simulink model "PMLSM_ThreeLoop_Simple"  (R2026a)
settings: Solver=FixedStepDiscrete  StopTime=12  FixedStep=PMLSM_Ts_s
InitFcn:
  | reload(get_param('PMLSM_ThreeLoop_Simple','ModelWorkspace'));
model workspace: external: MATLAB File init_PMLSM_ThreeLoop_Simple.m (data not in the file)
values from neighbouring files (symbols this model uses):
  CPU_Clock = 200e6    (= 200000000)    [PMSLM_Init_Params_MBDL4.m]    (also in init_PMLSM_ThreeLoop_Simple.m)
  Host_Enable_Schedule = [0 1 1 1]    [init_PMLSM_ThreeLoop_Simple.m]
  Host_Id_A = 0    [init_PMLSM_ThreeLoop_Simple.m]
  Host_Iq_A = 0    [init_PMLSM_ThreeLoop_Simple.m]
  Host_Iq_Test_Mode = 0    [init_PMLSM_ThreeLoop_Simple.m]
  Host_Load_N = 0    [init_PMLSM_ThreeLoop_Simple.m]
  Host_PI_Reset_EN = 0    [init_PMLSM_ThreeLoop_Simple.m]
  Host_Speed_mmps = 0    [init_PMLSM_ThreeLoop_Simple.m]
  Host_Speed_Ramp_s = 1    [init_PMLSM_ThreeLoop_Simple.m]
  Host_Start_s = 0.5    [init_PMLSM_ThreeLoop_Simple.m]
  Host_Target_mm = 100    [init_PMLSM_ThreeLoop_Simple.m]
  Host_Traj_Amax = 100    [init_PMLSM_ThreeLoop_Simple.m]
  Host_Traj_Jmax = 1000    [init_PMLSM_ThreeLoop_Simple.m]
  Host_Traj_Vmax = 20    [init_PMLSM_ThreeLoop_Simple.m]
  Iq_fric_run = 0.05    [PMSLM_Init_Params_MBDL4.m]
  Iq_fric_start = 0.40    (= 0.4)    [PMSLM_Init_Params_MBDL4.m]
  Iq_int_limit = 0.10    (= 0.1)    [PMSLM_Init_Params_MBDL4.m]    (also in init_PMLSM_ThreeLoop_Simple.m = 0.5)
  Kaw_d = Kaw_q    (= 0.2)    [PMSLM_Init_Params_MBDL4.m]    (also in init_PMLSM_ThreeLoop_Simple.m = Tuning_Gains.Kaw_d)
  Kaw_q = 0.2    [PMSLM_Init_Params_MBDL4.m]    (also in init_PMLSM_ThreeLoop_Simple.m = Tuning_Gains.Kaw_q)
  Kaw_s = 0.4    [PMSLM_Init_Params_MBDL4.m]    (also in init_PMLSM_ThreeLoop_Simple.m = Tuning_Gains.Kaw_s)
  Ki_ACR = ACR_Commissioning_Scale*Ki_ACR_Baseline    (= 2962.5)    [PMSLM_Init_Params_MBDL4.m]    (also in init_PMLSM_ThreeLoop_Simple.m = Tuning_Gains.Ki_ACR; init_PMLSM_mil_test_params.m = Kp_ACR*PMLSM_Rs_ohm/PMLSM_Lq_H)
  Ki_ASR = 0.05    [PMSLM_Init_Params_MBDL4.m]    (also in init_PMLSM_ThreeLoop_Simple.m = Tuning_Gains.Ki_ASR)
  Kp_ACR = ACR_Commissioning_Scale*Kp_ACR_Baseline    (= 2.18125)    [PMSLM_Init_Params_MBDL4.m]    (also in init_PMLSM_ThreeLoop_Simple.m = Tuning_Gains.Kp_ACR; init_PMLSM_mil_test_params.m = PMLSM_Lq_H/(4*MIL_AUM3S4_Current_PI_xi^2*MIL_AUM3S4_Current_)
  Kp_ASR = 0.03    [PMSLM_Init_Params_MBDL4.m]    (also in init_PMLSM_ThreeLoop_Simple.m = Tuning_Gains.Kp_ASR)
  Kp_pos = 5    [PMSLM_Init_Params_MBDL4.m]    (also in init_PMLSM_ThreeLoop_Simple.m = Tuning_Gains.Kp_pos)
  PMLSM_Bv_N_per_mps = 0    [init_PMLSM_ThreeLoop_Simple.m]    (also in init_PMLSM_plant_params.m)
  PMLSM_deadtime_current_eps_A = 1e-4    (= 0.0001)    [init_PMLSM_ThreeLoop_Simple.m]    (also in init_PMLSM_plant_params.m)
  PMLSM_deadtime_ratio = PMLSM_deadtime_s/Ts    (= 0.01)    [init_PMLSM_ThreeLoop_Simple.m]    (also in init_PMLSM_plant_params.m)
  PMLSM_Fc_N = 0    [init_PMLSM_ThreeLoop_Simple.m]    (also in init_PMLSM_plant_params.m)
  PMLSM_Kf_peak_N_per_Apeak = 31.4/sqrt(2)    [init_PMLSM_ThreeLoop_Simple.m]    (also in init_PMLSM_plant_params.m = PMLSM_Kf_rms_N_per_Arms/sqrt(2))
  PMLSM_Ld_H = Ld    (= 0.001745)    [PMSLM_Init_Params_MBDL4.m]    (also in init_PMLSM_ThreeLoop_Simple.m; init_PMLSM_plant_params.m)
  PMLSM_Lq_H = Lq    (= 0.001745)    [PMSLM_Init_Params_MBDL4.m]    (also in init_PMLSM_ThreeLoop_Simple.m; init_PMLSM_plant_params.m)
  PMLSM_M_kg = 0.91    [init_PMLSM_ThreeLoop_Simple.m]    (also in init_PMLSM_plant_params.m)
  PMLSM_psi_f_Wb = flux    (= 0.141)    [PMSLM_Init_Params_MBDL4.m]    (also in init_PMLSM_ThreeLoop_Simple.m; init_PMLSM_plant_params.m)
  PMLSM_pwm_period_counts = CPU_Clock*Ts/2    (= 10000)    [init_PMLSM_ThreeLoop_Simple.m]    (also in init_PMLSM_plant_params.m = 7500)
  PMLSM_Rs_ohm = Rs    (= 2.37)    [PMSLM_Init_Params_MBDL4.m]    (also in init_PMLSM_ThreeLoop_Simple.m; init_PMLSM_plant_params.m)
  PMLSM_tau_NN_m = 0.06    [init_PMLSM_ThreeLoop_Simple.m]    (also in init_PMLSM_plant_params.m)
  PMLSM_theta_offset_rad = 0    [init_PMLSM_ThreeLoop_Simple.m]    (also in init_PMLSM_plant_params.m)
  PMLSM_Ts_s = Ts/2    (= 5e-05)    [init_PMLSM_ThreeLoop_Simple.m]    (also in init_PMLSM_plant_params.m = 0.0001)
  PMLSM_v_eps_mps = 1e-3    (= 0.001)    [init_PMLSM_ThreeLoop_Simple.m]    (also in init_PMLSM_plant_params.m)
  Pos_deadband = 0.02    [PMSLM_Init_Params_MBDL4.m]    (also in init_PMLSM_ThreeLoop_Simple.m)
  Speed_loop_Iq_Limit = Iq_Limit    (= 0.3)    [PMSLM_Init_Params_MBDL4.m]    (also in init_PMLSM_ThreeLoop_Simple.m = 1)
  Ts = 1 / PWM_Freq    (= 0.0001)    [PMSLM_Init_Params_MBDL4.m]    (also in init_PMLSM_ThreeLoop_Simple.m)
  Ts_ACR = 1e-4    (= 0.0001)    [PMSLM_Init_Params_MBDL4.m]    (also in init_PMLSM_ThreeLoop_Simple.m)
  Ts_ASR = 1e-3    (= 0.001)    [PMSLM_Init_Params_MBDL4.m]    (also in init_PMLSM_ThreeLoop_Simple.m)
  Udc = 48    [PMSLM_Init_Params_MBDL4.m]    (also in init_PMLSM_ThreeLoop_Simple.m; init_PMLSM_mil_test_params.m)
  v_ff_eps = 0.5    [PMSLM_Init_Params_MBDL4.m]    (also in init_PMLSM_ThreeLoop_Simple.m)
  v_over_eps = 3    [PMSLM_Init_Params_MBDL4.m]    (also in init_PMLSM_ThreeLoop_Simple.m)
  V_pos_max_mmps = 10    [PMSLM_Init_Params_MBDL4.m]    (also in init_PMLSM_ThreeLoop_Simple.m = 20)
  v_ref_max = 20    [PMSLM_Init_Params_MBDL4.m]    (also in init_PMLSM_ThreeLoop_Simple.m)
  v_ref_set_step_dn = v_ref_set_rate_dn * Ts    (= 0.005)    [PMSLM_Init_Params_MBDL4.m]    (also in init_PMLSM_ThreeLoop_Simple.m)
  v_ref_set_step_up = v_ref_set_rate_up * Ts    (= 0.005)    [PMSLM_Init_Params_MBDL4.m]    (also in init_PMLSM_ThreeLoop_Simple.m)
  v_ref_zero_eps = 0.2    [PMSLM_Init_Params_MBDL4.m]    (also in init_PMLSM_ThreeLoop_Simple.m = 0)
  v_stick_off = 3.0    (= 3)    [PMSLM_Init_Params_MBDL4.m]
  v_stick_on = 1.0    (= 1)    [PMSLM_Init_Params_MBDL4.m]
undefined symbols (not defined in the file or in its folder): DiscIntNeverNeededParam
libraries: simulink x7, mcbeeMathTransformLib x2
settings Model: Creator=lww  LastModifiedBy=lww

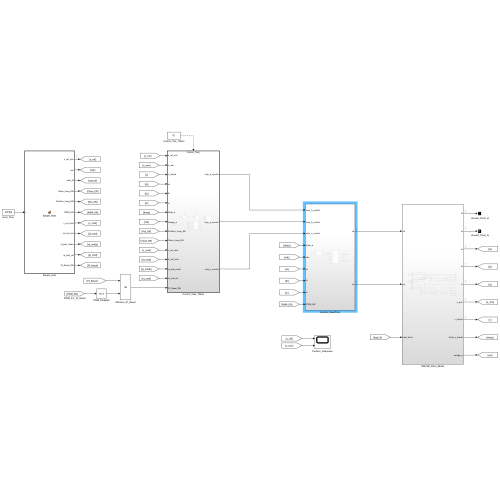
[thumbnail: Simulink's stored preview of the top-level diagram]
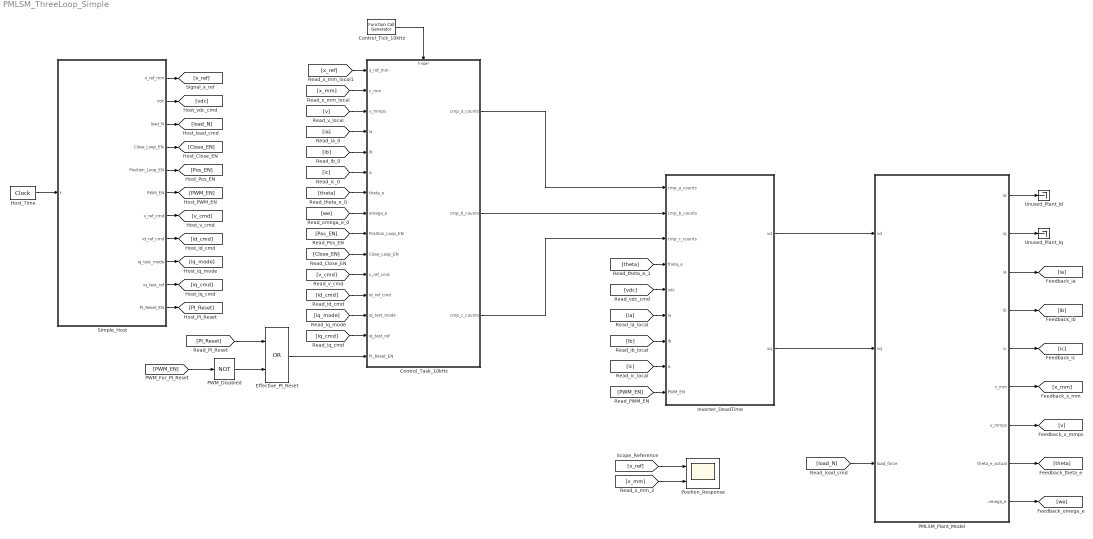
== system PMLSM_ThreeLoop_Simple ==
  Control_Task_10kHz : Subsystem
  Control_Tick_10kHz : FunctionCallGenerator  SampleTime=Ts
  Effective_PI_Reset : Logic  Operator=OR  AllPortsSameDT=off  OutDataTypeStr=boolean
  Host_Time : DigitalClock  SampleTime=Ts_ACR
  Inverter_DeadTime : Subsystem
  PMLSM_Plant_Model : Subsystem
  PWM_Disabled : Logic  Operator=NOT  AllPortsSameDT=off  OutDataTypeStr=boolean
  Position_Response : Scope  NumInputPorts=2
  Simple_Host : MATLAB Function  TreatAsAtomicUnit=on
  Unused_Plant_Id : Terminator
  Unused_Plant_Iq : Terminator
  wires:
  Host_Time/1 -> Simple_Host/1(t)
  [x_ref] -> Position_Response/1
  [ic] -> Inverter_DeadTime/8(ic)
  [ib] -> Inverter_DeadTime/7(ib)
  [ia] -> Inverter_DeadTime/6(ia)
  [x_mm] -> Position_Response/2
  [theta] -> Inverter_DeadTime/4(theta_e)
  [load_N] -> PMLSM_Plant_Model/3(load_force)
  [vdc] -> Inverter_DeadTime/5(vdc)
  Simple_Host/2(vdc) -> [vdc]
  Inverter_DeadTime/1(vd) -> PMLSM_Plant_Model/1(vd)
  Inverter_DeadTime/2(vq) -> PMLSM_Plant_Model/2(vq)
  PMLSM_Plant_Model/2(iq) -> Unused_Plant_Iq/1
  PMLSM_Plant_Model/1(id) -> Unused_Plant_Id/1
  PMLSM_Plant_Model/9(omega_e) -> [we]
  PMLSM_Plant_Model/8(theta_e_actual) -> [theta]
  PMLSM_Plant_Model/5(ic) -> [ic]
  PMLSM_Plant_Model/4(ib) -> [ib]
  PMLSM_Plant_Model/3(ia) -> [ia]
  PMLSM_Plant_Model/7(v_mmps) -> [v]
  PMLSM_Plant_Model/6(x_mm) -> [x_mm]
  Simple_Host/3(load_N) -> [load_N]
  Simple_Host/11(PI_Reset_EN) -> [PI_Reset]
  Simple_Host/10(iq_test_ref) -> [iq_cmd]
  Simple_Host/9(iq_test_mode) -> [iq_mode]
  Simple_Host/8(id_ref_cmd) -> [id_cmd]
  Simple_Host/7(v_ref_cmd) -> [v_cmd]
  [PWM_EN] -> Inverter_DeadTime/9(PWM_EN)
  Simple_Host/6(PWM_EN) -> [PWM_EN]
  Simple_Host/5(Position_Loop_EN) -> [Pos_EN]
  Simple_Host/4(Close_Loop_EN) -> [Close_EN]
  [PWM_EN] -> PWM_Disabled/1
  PWM_Disabled/1 -> Effective_PI_Reset/2
  Effective_PI_Reset/1 -> Control_Task_10kHz/15(PI_Reset_EN)
  [Close_EN] -> Control_Task_10kHz/10(Close_Loop_EN)
  [Pos_EN] -> Control_Task_10kHz/9(Position_Loop_EN)
  [v_cmd] -> Control_Task_10kHz/11(v_ref_cmd)
  [id_cmd] -> Control_Task_10kHz/12(id_ref_cmd)
  [iq_mode] -> Control_Task_10kHz/13(iq_test_mode)
  [iq_cmd] -> Control_Task_10kHz/14(iq_test_ref)
  [PI_Reset] -> Effective_PI_Reset/1
  Simple_Host/1(x_ref_mm) -> [x_ref]
  Control_Task_10kHz/1(cmp_a_counts) -> Inverter_DeadTime/1(cmp_a_counts)
  Control_Task_10kHz/2(cmp_b_counts) -> Inverter_DeadTime/2(cmp_b_counts)
  Control_Task_10kHz/3(cmp_c_counts) -> Inverter_DeadTime/3(cmp_c_counts)
  [x_mm] -> Control_Task_10kHz/2(x_mm)
  [v] -> Control_Task_10kHz/3(v_mmps)
  [ia] -> Control_Task_10kHz/4(ia)
  [ib] -> Control_Task_10kHz/5(ib)
  [ic] -> Control_Task_10kHz/6(ic)
  [we] -> Control_Task_10kHz/8(omega_e)
  [theta] -> Control_Task_10kHz/7(theta_e)
  Control_Tick_10kHz/1 -> Control_Task_10kHz/Trigger
  [x_ref] -> Control_Task_10kHz/1(x_ref_mm)

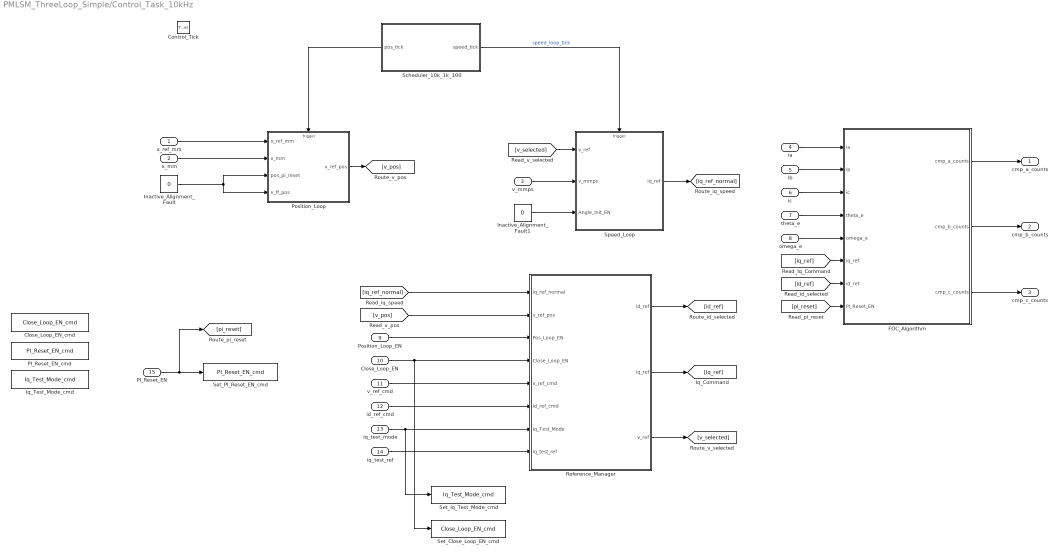
== system PMLSM_ThreeLoop_Simple/Control_Task_10kHz ==
  x_ref_mm : Inport
  x_mm : Inport  Port=2
  v_mmps : Inport  Port=3
  ia : Inport  Port=4
  ib : Inport  Port=5
  ic : Inport  Port=6
  theta_e : Inport  Port=7
  omega_e : Inport  Port=8
  Position_Loop_EN : Inport  Port=9
  Close_Loop_EN : Inport  Port=10
  v_ref_cmd : Inport  Port=11
  id_ref_cmd : Inport  Port=12
  iq_test_mode : Inport  Port=13
  iq_test_ref : Inport  Port=14
  PI_Reset_EN : Inport  Port=15
  Control_Tick : TriggerPort  TriggerType=function-call  VariantControl=(inherit)  PortDimensions=1
  Close_Loop_EN_cmd : DataStoreMemory  DataStoreName=Close_Loop_EN_cmd  WriteAfterWriteMsg=warning  InitialValue=1  ShowAdditionalParam=off
  FOC_Algorithm : Subsystem
  Inactive_Alignment_Fault : Constant  Value=0
  Inactive_Alignment_Fault1 : Constant  Value=0
  Iq_Test_Mode_cmd : DataStoreMemory  DataStoreName=Iq_Test_Mode_cmd  WriteAfterWriteMsg=warning  ShowAdditionalParam=off
  PI_Reset_EN_cmd : DataStoreMemory  DataStoreName=PI_Reset_EN_cmd  WriteAfterWriteMsg=warning  ShowAdditionalParam=off
  Position_Loop : Subsystem  TreatAsAtomicUnit=on
  Reference_Manager : Subsystem
  Scheduler_10k_1k_100 : Subsystem
      settings: PortSchema="{\"entries\":[{\"content\":{\"sides\":[{\"content\":{\"connectorIds\":[\"Out2\"]},\"type\":\"ConnectorPlacement.EquallySpacedRectSide\",\"uuid\":\"7a2cd2ad-1b6d-4ced-b4c0-dea2e76e4441\"},{\"content\":{\"connectorIds\":[\"Out1\"],\"side\":\"RIGHT\"},\"type\":\"ConnectorPlacement.EquallySpacedRectSide\",\"uuid\":\"f7db3b94-1126-4089-83bd-8e57d20e6fd7\"},{\"content\":{\"side\":\"TOP\"},\"type\":\"ConnectorPlacement.EquallySpacedRectSide\",\"uuid\":\"9153f6b5-22af-48be-92c0-68be43f93648\"}]},\"type\":\"ConnectorPlacement.EquallySpacedConnector\",\"uuid\":\"029fb485-bddc-4cd2-9c64-7547c8dffd2b\"}],\"packageUris\":[\"http://schema.mathworks.com/mf0/Connector/R2020b\"],\"version\":\"1.0\"}"
  Set_Close_Loop_EN_cmd : DataStoreWrite  Priority=-10  DataStoreName=Close_Loop_EN_cmd  IndexOptions=Index vector (dialog)  Indices=1  OutputSizes=1
  Set_Iq_Test_Mode_cmd : DataStoreWrite  Priority=-10  DataStoreName=Iq_Test_Mode_cmd  IndexOptions=Index vector (dialog)  Indices=1  OutputSizes=1
  Set_PI_Reset_EN_cmd : DataStoreWrite  Priority=-10  DataStoreName=PI_Reset_EN_cmd  IndexOptions=Index vector (dialog)  Indices=1  OutputSizes=1
  Speed_Loop : Subsystem  TreatAsAtomicUnit=on
  cmp_a_counts : Outport
  cmp_b_counts : Outport  Port=2
  cmp_c_counts : Outport  Port=3
  wires:
  [iq_ref] -> FOC_Algorithm/6(iq_ref)
  FOC_Algorithm/3(cmp_c_counts) -> cmp_c_counts/1
  FOC_Algorithm/2(cmp_b_counts) -> cmp_b_counts/1
  FOC_Algorithm/1(cmp_a_counts) -> cmp_a_counts/1
  omega_e/1 -> FOC_Algorithm/5(omega_e)
  theta_e/1 -> FOC_Algorithm/4(theta_e)
  ic/1 -> FOC_Algorithm/3(ic)
  ib/1 -> FOC_Algorithm/2(ib)
  ia/1 -> FOC_Algorithm/1(ia)
  Reference_Manager/2(iq_ref) -> [iq_ref]
  iq_test_ref/1 -> Reference_Manager/8(iq_test_ref)
  id_ref_cmd/1 -> Reference_Manager/6(id_ref_cmd)
  v_ref_cmd/1 -> Reference_Manager/5(v_ref_cmd)
  Position_Loop_EN/1 -> Reference_Manager/3(Pos_Loop_EN)
  [pi_reset] -> FOC_Algorithm/8(PI_Reset_EN)
  [id_ref] -> FOC_Algorithm/7(id_ref)
  [v_selected] -> Speed_Loop/1(v_ref)
  [iq_ref_normal] -> Reference_Manager/1(iq_ref_normal)
  [v_pos] -> Reference_Manager/2(v_ref_pos)
  Reference_Manager/3(v_ref) -> [v_selected]
  Inactive_Alignment_Fault/1 -> Position_Loop/3(pos_pi_reset), Position_Loop/4(v_ff_pos)
  Speed_Loop/1(iq_ref) -> [iq_ref_normal]
  Position_Loop/1(v_ref_pos) -> [v_pos]
  x_mm/1 -> Position_Loop/2(x_mm)
  x_ref_mm/1 -> Position_Loop/1(x_ref_mm)
  Scheduler_10k_1k_100/1(speed_tick) -> Speed_Loop/Trigger  "speed_loop_tick"
  Scheduler_10k_1k_100/2(pos_tick) -> Position_Loop/Trigger
  PI_Reset_EN/1 -> [pi_reset], Set_PI_Reset_EN_cmd/1
  Reference_Manager/1(id_ref) -> [id_ref]
  iq_test_mode/1 -> Set_Iq_Test_Mode_cmd/1, Reference_Manager/7(Iq_Test_Mode)
  Close_Loop_EN/1 -> Set_Close_Loop_EN_cmd/1, Reference_Manager/4(Close_Loop_EN)
  Inactive_Alignment_Fault1/1 -> Speed_Loop/3(Angle_Init_EN)
  v_mmps/1 -> Speed_Loop/2(v_mmps)

== system PMLSM_ThreeLoop_Simple/Inverter_DeadTime ==
  note: 死区时间建立
  note: 半拍更新延迟
  cmp_a_counts : Inport
  cmp_b_counts : Inport  Port=2
  cmp_c_counts : Inport  Port=3
  theta_e : Inport  Port=4
  vdc : Inport  Port=5
  ia : Inport  Port=6
  ib : Inport  Port=7
  ic : Inport  Port=8
  PWM_EN : Inport  Port=9
  DeadTime_Voltage_Model : Subsystem
  PWM_Update_HalfTs : Subsystem
  vd_PWM_Enable : Product  Inputs=**
  vq_PWM_Enable : Product  Inputs=**
  vd : Outport
  vq : Outport  Port=2
  wires:
  cmp_c_counts/1 -> PWM_Update_HalfTs/3(duty_c)
  cmp_b_counts/1 -> PWM_Update_HalfTs/2(duty_b)
  cmp_a_counts/1 -> PWM_Update_HalfTs/1(duty_a)
  vq_PWM_Enable/1 -> vq/1
  vd_PWM_Enable/1 -> vd/1
  PWM_Update_HalfTs/1(duty_a_delayed) -> DeadTime_Voltage_Model/1(duty_a)
  PWM_Update_HalfTs/2(duty_b_delayed) -> DeadTime_Voltage_Model/2(duty_b)
  PWM_Update_HalfTs/3(duty_c_delayed) -> DeadTime_Voltage_Model/3(duty_c)
  theta_e/1 -> DeadTime_Voltage_Model/4(theta_e)
  vdc/1 -> DeadTime_Voltage_Model/5(vdc)
  ia/1 -> DeadTime_Voltage_Model/6(ia_phase)
  ib/1 -> DeadTime_Voltage_Model/7(ib_phase)
  ic/1 -> DeadTime_Voltage_Model/8(ic_phase)
  DeadTime_Voltage_Model/1(vd_from_duty) -> vd_PWM_Enable/1
  DeadTime_Voltage_Model/2(vq_from_duty) -> vq_PWM_Enable/1
  PWM_EN/1 -> vd_PWM_Enable/2, vq_PWM_Enable/2

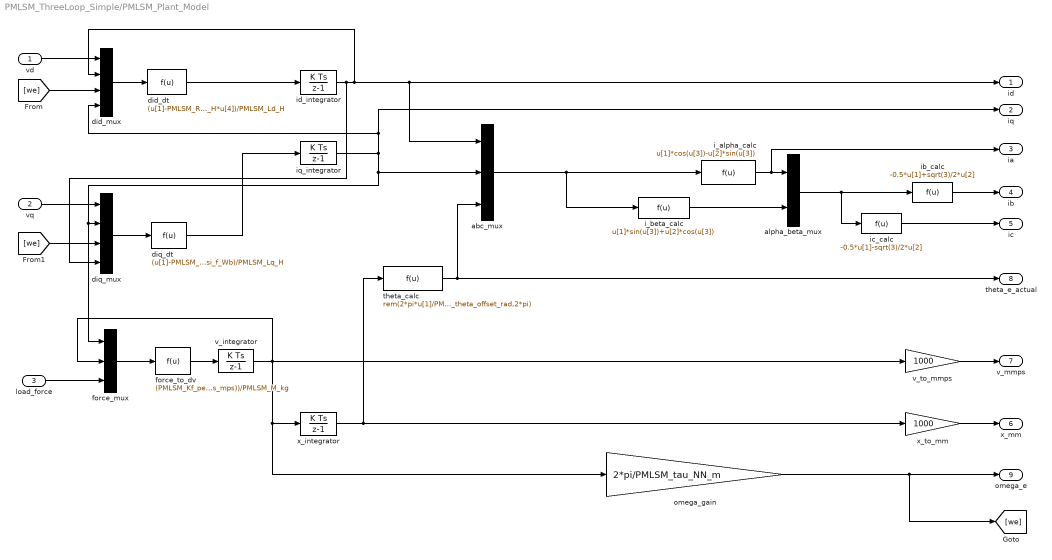
== system PMLSM_ThreeLoop_Simple/PMLSM_Plant_Model ==
  vd : Inport
  vq : Inport  Port=2
  load_force : Inport  Port=3
  abc_mux : Mux  Inputs=3
  alpha_beta_mux : Mux  Inputs=2
  did_dt : Fcn  Expr=(u[1]-PMLSM_Rs_ohm*u[2]+u[3]*PMLSM_Lq_H*u[4])/PMLSM_Ld_H
  did_mux : Mux
  diq_dt : Fcn  Expr=(u[1]-PMLSM_Rs_ohm*u[2]-u[3]*PMLSM_Ld_H*u[4]-u[3]*PMLSM_psi_f_Wb)/PMLSM_Lq_H
  diq_mux : Mux
  force_mux : Mux  Inputs=3
  force_to_dv : Fcn  Expr=(PMLSM_Kf_peak_N_per_Apeak*u[1]-u[3]-PMLSM_Bv_N_per_mps*u[2]-PMLSM_Fc_N*tanh(u[2]/PMLSM_v_eps_mps))/PMLSM_M_kg
  i_alpha_calc : Fcn  Expr=u[1]*cos(u[3])-u[2]*sin(u[3])
  i_beta_calc : Fcn  Expr=u[1]*sin(u[3])+u[2]*cos(u[3])
  ib_calc : Fcn  Expr=-0.5*u[1]+sqrt(3)/2*u[2]
  ic_calc : Fcn  Expr=-0.5*u[1]-sqrt(3)/2*u[2]
  id_integrator : DiscreteIntegrator  gainval=1  SampleTime=PMLSM_Ts_s  ICPrevOutput=DiscIntNeverNeededParam  ICPrevScaledInput=DiscIntNeverNeededParam
  iq_integrator : DiscreteIntegrator  gainval=1  SampleTime=PMLSM_Ts_s  ICPrevOutput=DiscIntNeverNeededParam  ICPrevScaledInput=DiscIntNeverNeededParam
  omega_gain : Gain  Gain=2*pi/PMLSM_tau_NN_m
  theta_calc : Fcn  Expr=rem(2*pi*u[1]/PMLSM_tau_NN_m+PMLSM_theta_offset_rad,2*pi)
  v_integrator : DiscreteIntegrator  gainval=1  SampleTime=PMLSM_Ts_s  ICPrevOutput=DiscIntNeverNeededParam  ICPrevScaledInput=DiscIntNeverNeededParam
  v_to_mmps : Gain  Gain=1000
  x_integrator : DiscreteIntegrator  gainval=1  SampleTime=PMLSM_Ts_s  ICPrevOutput=DiscIntNeverNeededParam  ICPrevScaledInput=DiscIntNeverNeededParam
  x_to_mm : Gain  Gain=1000
  id : Outport
  iq : Outport  Port=2
  ia : Outport  Port=3
  ib : Outport  Port=4
  ic : Outport  Port=5
  x_mm : Outport  Port=6
  v_mmps : Outport  Port=7
  theta_e_actual : Outport  Port=8
  omega_e : Outport  Port=9
  wires:
  ic_calc/1 -> ic/1
  ib_calc/1 -> ib/1
  alpha_beta_mux/1 -> ic_calc/1, ib_calc/1
  i_beta_calc/1 -> alpha_beta_mux/2
  i_alpha_calc/1 -> alpha_beta_mux/1, ia/1
  force_to_dv/1 -> v_integrator/1
  force_mux/1 -> force_to_dv/1
  load_force/1 -> force_mux/3
  diq_dt/1 -> iq_integrator/1
  diq_mux/1 -> diq_dt/1
  vq/1 -> diq_mux/1
  did_dt/1 -> id_integrator/1
  did_mux/1 -> did_dt/1
  vd/1 -> did_mux/1
  x_to_mm/1 -> x_mm/1
  v_to_mmps/1 -> v_mmps/1
  theta_calc/1 -> theta_e_actual/1, abc_mux/3
  omega_gain/1 -> [we], omega_e/1
  id_integrator/1 -> id/1, abc_mux/1, did_mux/2, diq_mux/4
  iq_integrator/1 -> abc_mux/2, force_mux/1, diq_mux/2, iq/1, did_mux/4
  v_integrator/1 -> omega_gain/1, x_integrator/1, v_to_mmps/1, force_mux/2
  x_integrator/1 -> theta_calc/1, x_to_mm/1
  abc_mux/1 -> i_alpha_calc/1, i_beta_calc/1
  [we] -> did_mux/3
  [we] -> diq_mux/3

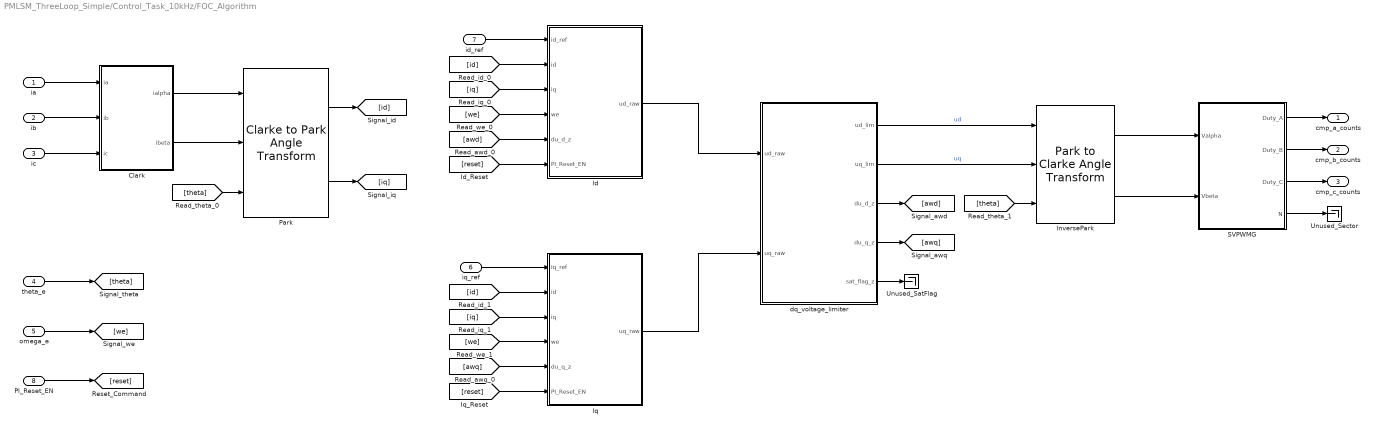
== system PMLSM_ThreeLoop_Simple/Control_Task_10kHz/FOC_Algorithm ==
  ia : Inport
  ib : Inport  Port=2
  ic : Inport  Port=3
  theta_e : Inport  Port=4
  omega_e : Inport  Port=5
  iq_ref : Inport  Port=6
  id_ref : Inport  Port=7
  PI_Reset_EN : Inport  Port=8
  Clark : Subsystem  TreatAsAtomicUnit=on  RTWFcnName=Clack_Fun
      settings: RTWFcnNameOpts=User specified
  Id : Subsystem  TreatAsAtomicUnit=on  RTWFcnName=Id_Fun
      settings: RTWFcnNameOpts=User specified
  InversePark : mcbeeMathTransformLib/Park to Clarke Angle Transform  AxisAlignment=D-axis  UseWithEmbedded=on  PhaseInput=Two inputs  ThetaInput=Electrical position  AngleInput=Radians  N_points=1024
      settings: LibrarySourceBlock=mcbhdllib/Controls/Math Transforms/Inverse Park Transform
  Iq : Subsystem  TreatAsAtomicUnit=on  RTWFcnName=Iq_Fun
      settings: RTWFcnNameOpts=User specified
  Park : mcbeeMathTransformLib/Clarke to Park Angle Transform  AxisAlignment=D-axis  UseWithEmbedded=on  PhaseInput=Two inputs  ThetaInput=Electrical position  AngleInput=Radians  N_points=1024
      settings: LibrarySourceBlock=mcblib/Controls/Math Transforms/Park Transform
  SVPWMG : Subsystem  TreatAsAtomicUnit=on  RTWFcnName=SVPWM_Gen_Fun
      settings: RTWFcnNameOpts=User specified
  Unused_SatFlag : Terminator
  Unused_Sector : Terminator
  dq_voltage_limiter : Subsystem
  cmp_a_counts : Outport
  cmp_b_counts : Outport  Port=2
  cmp_c_counts : Outport  Port=3
  wires:
  SVPWMG/4("N ") -> Unused_Sector/1
  SVPWMG/3(Duty_C) -> cmp_c_counts/1
  SVPWMG/2(Duty_B) -> cmp_b_counts/1
  SVPWMG/1(Duty_A) -> cmp_a_counts/1
  ic/1 -> Clark/3(ic)
  ib/1 -> Clark/2(ib)
  ia/1 -> Clark/1(ia)
  [theta] -> InversePark/3
  [theta] -> Park/3
  Clark/1(ialpha) -> Park/1
  Clark/2(ibeta) -> Park/2
  theta_e/1 -> [theta]
  Park/1 -> [id]
  Park/2 -> [iq]
  omega_e/1 -> [we]
  dq_voltage_limiter/3(du_d_z) -> [awd]
  dq_voltage_limiter/4(du_q_z) -> [awq]
  dq_voltage_limiter/5(sat_flag_z) -> Unused_SatFlag/1
  dq_voltage_limiter/1(ud_lim) -> InversePark/1  "ud"
  dq_voltage_limiter/2(uq_lim) -> InversePark/2  "uq"
  InversePark/1 -> SVPWMG/1(Valpha)
  InversePark/2 -> SVPWMG/2(Vbeta)
  [reset] -> Iq/6(PI_Reset_EN)
  [reset] -> Id/6(PI_Reset_EN)
  id_ref/1 -> Id/1(id_ref)
  PI_Reset_EN/1 -> [reset]
  Iq/1(uq_raw) -> dq_voltage_limiter/2(uq_raw)
  Id/1(ud_raw) -> dq_voltage_limiter/1(ud_raw)
  iq_ref/1 -> Iq/1(Iq_ref)
  [id] -> Id/2(id)
  [id] -> Iq/2(id)
  [iq] -> Id/3(iq)
  [iq] -> Iq/3(iq)
  [we] -> Id/4(we)
  [we] -> Iq/4(we)
  [awd] -> Id/5(du_d_z)
  [awq] -> Iq/5(du_q_z)

== system PMLSM_ThreeLoop_Simple/Control_Task_10kHz/Position_Loop ==
  x_ref_mm : Inport
  x_mm : Inport  Port=2
  pos_pi_reset : Inport  Port=3
  v_ff_pos : Inport  Port=4
  Trigger : TriggerPort  VariantControl=(inherit)
  Dead Zone : DeadZone  LowerValue=-Pos_deadband  UpperValue=+Pos_deadband
  Gain : Gain  Gain=Kp_pos
  Saturation : Saturate  UpperLimit=V_pos_max_mmps  LowerLimit=-V_pos_max_mmps
  Sum : Sum  Inputs=|+-
  Sum1 : Sum  Inputs=|++
  Terminator : Terminator
  v_ref_pos : Outport
  wires:
  x_ref_mm/1 -> Sum/1
  x_mm/1 -> Sum/2
  Sum/1 -> Dead Zone/1  "e_pos"
  Dead Zone/1 -> Gain/1
  Gain/1 -> Sum1/1
  v_ff_pos/1 -> Sum1/2
  Sum1/1 -> Saturation/1
  pos_pi_reset/1 -> Terminator/1
  Saturation/1 -> v_ref_pos/1  "obs_v_ref_pos"

== system PMLSM_ThreeLoop_Simple/Control_Task_10kHz/Reference_Manager ==
  iq_ref_normal : Inport
  v_ref_pos : Inport  Port=2
  Pos_Loop_EN : Inport  Port=3
  Close_Loop_EN : Inport  Port=4
  v_ref_cmd : Inport  Port=5
  id_ref_cmd : Inport  Port=6
  Iq_Test_Mode : Inport  Port=7
  iq_test_ref : Inport  Port=8
  Constant15 : Constant  Value=0
  Saturation : Saturate  UpperLimit=v_ref_max  LowerLimit=-v_ref_max
  Switch : Switch  Criteria=u2 > Threshold  Threshold=0.5  SaturateOnIntegerOverflow=off  InputSameDT=off
  Switch9 : Switch  Criteria=u2 > Threshold  Threshold=0.5  SaturateOnIntegerOverflow=off  InputSameDT=off
  v_ref_closed_sel : Switch  Criteria=u2 > Threshold  Threshold=0.5  SaturateOnIntegerOverflow=off  InputSameDT=off
  v_ref_set_slew_limiter : Subsystem
  id_ref : Outport
  iq_ref : Outport  Port=2
  v_ref : Outport  Port=3
  wires:
  Switch/1 -> iq_ref/1
  Switch9/1 -> v_ref/1
  Close_Loop_EN/1 -> Switch9/2
  iq_test_ref/1 -> Switch/1
  Iq_Test_Mode/1 -> Switch/2
  Constant15/1 -> Switch9/3
  iq_ref_normal/1 -> Switch/3
  id_ref_cmd/1 -> id_ref/1
  v_ref_set_slew_limiter/1(v_ref_set_limited) -> Saturation/1
  v_ref_pos/1 -> v_ref_closed_sel/1
  v_ref_closed_sel/1 -> v_ref_set_slew_limiter/1(v_ref_set)  "v_ref_closed"
  Pos_Loop_EN/1 -> v_ref_closed_sel/2
  Saturation/1 -> Switch9/1
  v_ref_cmd/1 -> v_ref_closed_sel/3

== system PMLSM_ThreeLoop_Simple/Control_Task_10kHz/Scheduler_10k_1k_100 ==
  note: position 计数链(/100)
  note: speed 计数链(/10)
  Add1 : Sum
  Add2 : Sum
  Constant1 : Constant
  Constant2 : Constant  Value=0
  Constant3 : Constant
  Constant4 : Constant  Value=0
  Logical Operator : Logic  AllPortsSameDT=off  OutDataTypeStr=boolean
  pos_cnt_hold_sel : Switch  Criteria=u2 > Threshold  Threshold=0.5  SaturateOnIntegerOverflow=off  InputSameDT=off
  pos_cnt_update_sel : Switch  Criteria=u2 > Threshold  Threshold=0.5  SaturateOnIntegerOverflow=off  InputSameDT=off
  pos_cnt_z : UnitDelay  SampleTime=-1
  pos_tc : simulink/Logic and Bit Operations/Compare To Constant  relop=>=  const=10  OutDataTypeStr=boolean
  spd_cnt_next_sel : Switch  Criteria=u2 > Threshold  Threshold=0.5  SaturateOnIntegerOverflow=off  InputSameDT=off
  spd_cnt_z : UnitDelay  SampleTime=-1
  spd_tc : simulink/Logic and Bit Operations/Compare To Constant  relop=>=  const=10  OutDataTypeStr=boolean
  speed_tick : Outport
  pos_tick : Outport  Port=2
  wires:
  spd_cnt_z/1 -> Add1/1
  spd_tc/1 -> speed_tick/1, Logical Operator/1, pos_cnt_hold_sel/2, spd_cnt_next_sel/2
  Constant1/1 -> Add1/2
  Constant2/1 -> spd_cnt_next_sel/1
  spd_cnt_next_sel/1 -> spd_cnt_z/1
  Add1/1 -> spd_cnt_next_sel/3, spd_tc/1  "spd_cnt_inc"
  pos_cnt_z/1 -> Add2/1, pos_cnt_hold_sel/3
  Constant3/1 -> Add2/2
  Add2/1 -> pos_cnt_update_sel/3, pos_tc/1  "pos_cnt_inc"
  pos_tc/1 -> Logical Operator/2, pos_cnt_update_sel/2
  Constant4/1 -> pos_cnt_update_sel/1
  pos_cnt_update_sel/1 -> pos_cnt_hold_sel/1  "pos_cnt_update_candidate"
  pos_cnt_hold_sel/1 -> pos_cnt_z/1
  Logical Operator/1 -> pos_tick/1

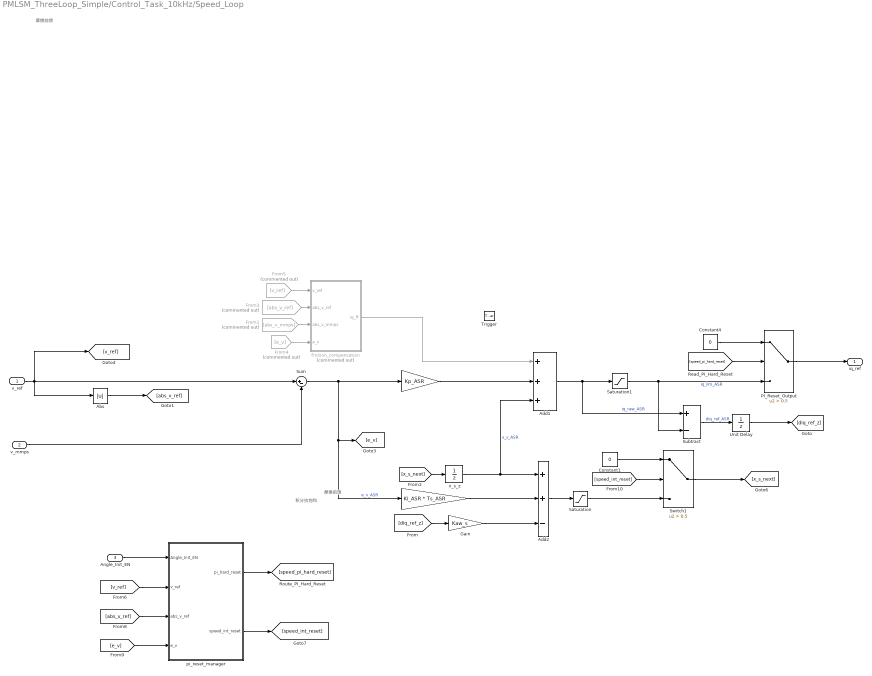
== system PMLSM_ThreeLoop_Simple/Control_Task_10kHz/Speed_Loop ==
  note: 摩擦前馈
  note: 积分抗饱和
  note: 摩擦前馈
  v_ref : Inport
  v_mmps : Inport  Port=2
  Angle_Init_EN : Inport  Port=3
  Trigger : TriggerPort  VariantControl=(inherit)
  " " : Gain  Gain=Ki_ASR * Ts_ASR
  "  " : Gain  Gain=Kp_ASR
  Abs : Abs  SaturateOnIntegerOverflow=off
  Add1 : Sum  Inputs=+++
  Add2 : Sum  Inputs=++-
  Constant1 : Constant  Value=0
  Constant4 : Constant  Value=0
  From1 : From  Commented=on  GotoTag=abs_v_mmps
  From3 : From  Commented=on  GotoTag=abs_v_ref
  From4 : From  Commented=on  GotoTag=e_v
  From5 : From  Commented=on  GotoTag=v_ref
  Gain : Gain  Gain=Kaw_s
  PI_Reset_Output : Switch  Criteria=u2 > Threshold  Threshold=0.5  SaturateOnIntegerOverflow=off  InputSameDT=off
  Saturation : Saturate  UpperLimit=Iq_int_limit  LowerLimit=-Iq_int_limit
  Saturation1 : Saturate  UpperLimit=Speed_loop_Iq_Limit  LowerLimit=-Speed_loop_Iq_Limit
  Subtract : Sum  Inputs=+-
  Sum : Sum  Inputs=|+-
  Switch1 : Switch  Criteria=u2 > Threshold  Threshold=0.5  SaturateOnIntegerOverflow=off  InputSameDT=off
  Unit Delay : UnitDelay  SampleTime=-1
  friction_compensation : Subsystem  Commented=on
  pi_reset_manager : Subsystem
  x_s_z : UnitDelay  SampleTime=-1
  iq_ref : Outport
  wires:
  Sum/1 -> [e_v], " "/1, "  "/1  "e_v_ASR"
  Add1/1 -> Subtract/1, Saturation1/1  "iq_raw_ASR"
  v_ref/1 -> Sum/1, Abs/1, [v_ref]
  Saturation1/1 -> PI_Reset_Output/3, Subtract/2  "iq_lim_ASR"
  [x_s_next] -> x_s_z/1
  Add2/1 -> Saturation/1
  Gain/1 -> Add2/3
  " "/1 -> Add2/2
  Subtract/1 -> Unit Delay/1  "diq_ref_ASR"
  Unit Delay/1 -> [diq_ref_z]
  [diq_ref_z] -> Gain/1
  Constant1/1 -> Switch1/1
  PI_Reset_Output/1 -> iq_ref/1
  Constant4/1 -> PI_Reset_Output/1
  "  "/1 -> Add1/2
  friction_compensation/1(iq_ff) -> Add1/1
  x_s_z/1 -> Add1/3, Add2/1  "x_s_ASR"
  From4/1 -> friction_compensation/4(e_v)
  From1/1 -> friction_compensation/3(abs_v_mmps)
  From3/1 -> friction_compensation/2(abs_v_ref)
  Abs/1 -> [abs_v_ref]
  Angle_Init_EN/1 -> pi_reset_manager/1(Angle_Init_EN)
  From5/1 -> friction_compensation/1(v_ref)
  [v_ref] -> pi_reset_manager/2(v_ref)
  [abs_v_ref] -> pi_reset_manager/3(abs_v_ref)
  [e_v] -> pi_reset_manager/4(e_v)
  [speed_pi_hard_reset] -> PI_Reset_Output/2
  pi_reset_manager/2(speed_int_reset) -> [speed_int_reset]
  pi_reset_manager/1(pi_hard_reset) -> [speed_pi_hard_reset]
  [speed_int_reset] -> Switch1/2
  Switch1/1 -> [x_s_next]
  Saturation/1 -> Switch1/3
  v_mmps/1 -> Sum/2

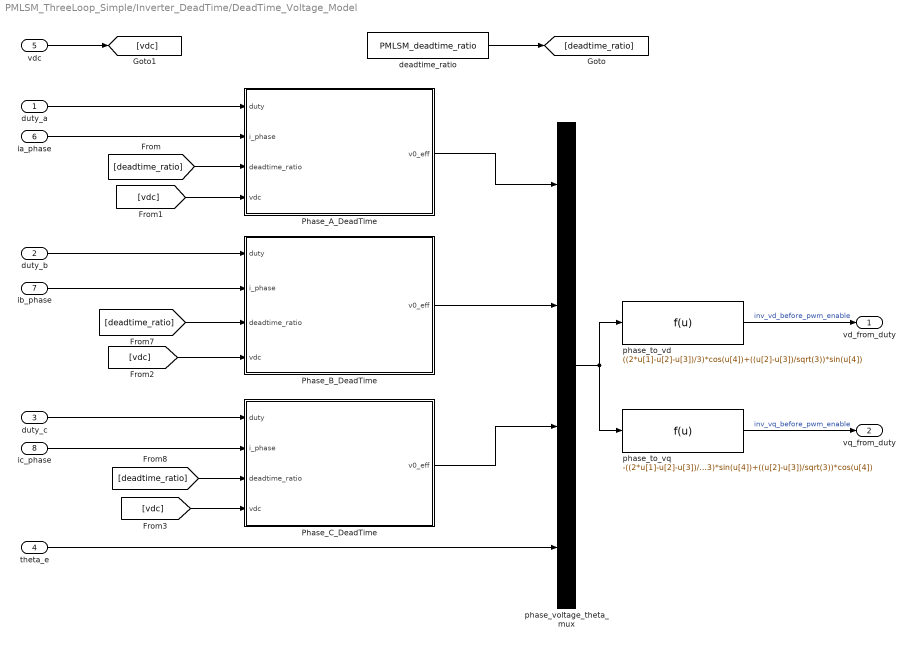
== system PMLSM_ThreeLoop_Simple/Inverter_DeadTime/DeadTime_Voltage_Model ==
  duty_a : Inport
  duty_b : Inport  Port=2
  duty_c : Inport  Port=3
  theta_e : Inport  Port=4
  vdc : Inport  Port=5
  ia_phase : Inport  Port=6
  ib_phase : Inport  Port=7
  ic_phase : Inport  Port=8
  Phase_A_DeadTime : Subsystem
  Phase_B_DeadTime : Subsystem
  Phase_C_DeadTime : Subsystem
  deadtime_ratio : Constant  Value=PMLSM_deadtime_ratio
  phase_to_vd : Fcn  Expr=((2*u[1]-u[2]-u[3])/3)*cos(u[4])+((u[2]-u[3])/sqrt(3))*sin(u[4])
  phase_to_vq : Fcn  Expr=-((2*u[1]-u[2]-u[3])/3)*sin(u[4])+((u[2]-u[3])/sqrt(3))*cos(u[4])
  phase_voltage_theta_mux : Mux
  vd_from_duty : Outport
  vq_from_duty : Outport  Port=2
  wires:
  [deadtime_ratio] -> Phase_C_DeadTime/3(deadtime_ratio)
  [deadtime_ratio] -> Phase_B_DeadTime/3(deadtime_ratio)
  [deadtime_ratio] -> Phase_A_DeadTime/3(deadtime_ratio)
  [vdc] -> Phase_C_DeadTime/4(vdc)
  [vdc] -> Phase_B_DeadTime/4(vdc)
  [vdc] -> Phase_A_DeadTime/4(vdc)
  vdc/1 -> [vdc]
  theta_e/1 -> phase_voltage_theta_mux/4
  Phase_C_DeadTime/1(v0_eff) -> phase_voltage_theta_mux/3
  Phase_B_DeadTime/1(v0_eff) -> phase_voltage_theta_mux/2
  Phase_A_DeadTime/1(v0_eff) -> phase_voltage_theta_mux/1
  ic_phase/1 -> Phase_C_DeadTime/2(i_phase)
  duty_c/1 -> Phase_C_DeadTime/1(duty)
  ib_phase/1 -> Phase_B_DeadTime/2(i_phase)
  duty_b/1 -> Phase_B_DeadTime/1(duty)
  ia_phase/1 -> Phase_A_DeadTime/2(i_phase)
  duty_a/1 -> Phase_A_DeadTime/1(duty)
  deadtime_ratio/1 -> [deadtime_ratio]
  phase_to_vq/1 -> vq_from_duty/1  "inv_vq_before_pwm_enable"
  phase_to_vd/1 -> vd_from_duty/1  "inv_vd_before_pwm_enable"
  phase_voltage_theta_mux/1 -> phase_to_vq/1, phase_to_vd/1

== system PMLSM_ThreeLoop_Simple/Inverter_DeadTime/PWM_Update_HalfTs ==
  duty_a : Inport
  duty_b : Inport  Port=2
  duty_c : Inport  Port=3
  a_cmd_zoh : ZeroOrderHold  SampleTime=Ts
  a_half_Ts : UnitDelay  InitialCondition=PMLSM_pwm_period_counts/2  SampleTime=Ts/2
  b_cmd_zoh : ZeroOrderHold  SampleTime=Ts
  b_half_Ts : UnitDelay  InitialCondition=PMLSM_pwm_period_counts/2  SampleTime=Ts/2
  c_cmd_zoh : ZeroOrderHold  SampleTime=Ts
  c_half_Ts : UnitDelay  InitialCondition=PMLSM_pwm_period_counts/2  SampleTime=Ts/2
  duty_a_delayed : Outport
  duty_b_delayed : Outport  Port=2
  duty_c_delayed : Outport  Port=3
  wires:
  duty_c/1 -> c_cmd_zoh/1
  duty_b/1 -> b_cmd_zoh/1
  duty_a/1 -> a_cmd_zoh/1
  c_half_Ts/1 -> duty_c_delayed/1
  b_half_Ts/1 -> duty_b_delayed/1
  a_half_Ts/1 -> duty_a_delayed/1
  a_cmd_zoh/1 -> a_half_Ts/1
  b_cmd_zoh/1 -> b_half_Ts/1
  c_cmd_zoh/1 -> c_half_Ts/1

== system PMLSM_ThreeLoop_Simple/Control_Task_10kHz/FOC_Algorithm/Clark ==
  note: alpha=(A-0.5*(B+C))*2/3
      | Beta=sqrt(3)/2*(B-C)*2/3
  ia : Inport
  ib : Inport  Port=2
  ic : Inport  Port=3
  Add : Sum  Inputs=+--
  Add1 : Sum  Inputs=+-
  Gain : Gain  Gain=0.5
  Gain1 : Gain  Gain=0.5
  Gain2 : Gain  Gain=2/3
  Gain3 : Gain  Gain=1/sqrt(3)
  ialpha : Outport
  ibeta : Outport  Port=2
  wires:
  Gain/1 -> Add/2
  Gain2/1 -> ialpha/1  "ialf"
  Add/1 -> Gain2/1
  Gain3/1 -> ibeta/1  "ibeta"
  ic/1 -> Gain1/1, Add1/2
  Add1/1 -> Gain3/1
  ib/1 -> Gain/1, Add1/1
  ia/1 -> Add/1
  Gain1/1 -> Add/3

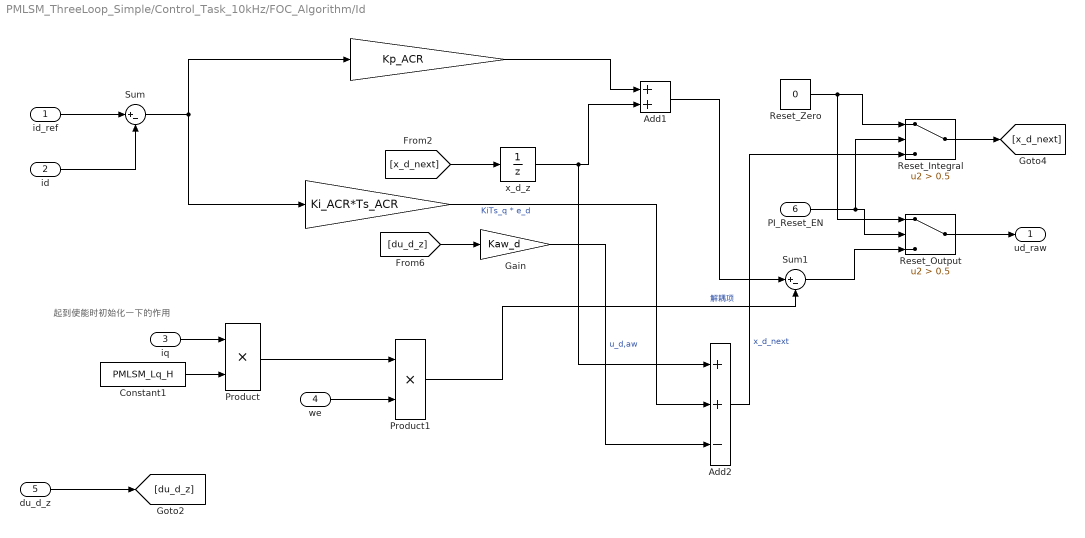
== system PMLSM_ThreeLoop_Simple/Control_Task_10kHz/FOC_Algorithm/Id ==
  note: 起到使能时初始化一下的作用
  id_ref : Inport
  id : Inport  Port=2
  iq : Inport  Port=3
  we : Inport  Port=4
  du_d_z : Inport  Port=5
  PI_Reset_EN : Inport  Port=6
  " " : Gain  Gain=Ki_ACR*Ts_ACR
  "  " : Gain  Gain=Kp_ACR
  Add1 : Sum
  Add2 : Sum  Inputs=++-
  Constant1 : Constant  Value=PMLSM_Lq_H
  Gain : Gain  Gain=Kaw_d
  Product : Product
  Product1 : Product
  Reset_Integral : Switch  Criteria=u2 > Threshold  Threshold=0.5  SaturateOnIntegerOverflow=off  InputSameDT=off
  Reset_Output : Switch  Criteria=u2 > Threshold  Threshold=0.5  SaturateOnIntegerOverflow=off  InputSameDT=off
  Reset_Zero : Constant  Value=0
  Sum : Sum  Inputs=|+-
  Sum1 : Sum  Inputs=|+-
  x_d_z : UnitDelay  SampleTime=-1
  ud_raw : Outport
  wires:
  [du_d_z] -> Gain/1
  [x_d_next] -> x_d_z/1
  du_d_z/1 -> [du_d_z]
  "  "/1 -> Add1/1
  Constant1/1 -> Product/2
  Product/1 -> Product1/1
  we/1 -> Product1/2
  Sum/1 -> "  "/1, " "/1
  id/1 -> Sum/2
  id_ref/1 -> Sum/1
  iq/1 -> Product/1
  Reset_Output/1 -> ud_raw/1
  Reset_Integral/1 -> [x_d_next]
  PI_Reset_EN/1 -> Reset_Output/2, Reset_Integral/2
  Reset_Zero/1 -> Reset_Output/1, Reset_Integral/1
  Add2/1 -> Reset_Integral/3  "x_d_next"
  Sum1/1 -> Reset_Output/3
  " "/1 -> Add2/2  "KiTs_q * e_d"
  Gain/1 -> Add2/3  "u_d,aw"
  x_d_z/1 -> Add2/1, Add1/2
  Add1/1 -> Sum1/1
  Product1/1 -> Sum1/2  "解耦项"

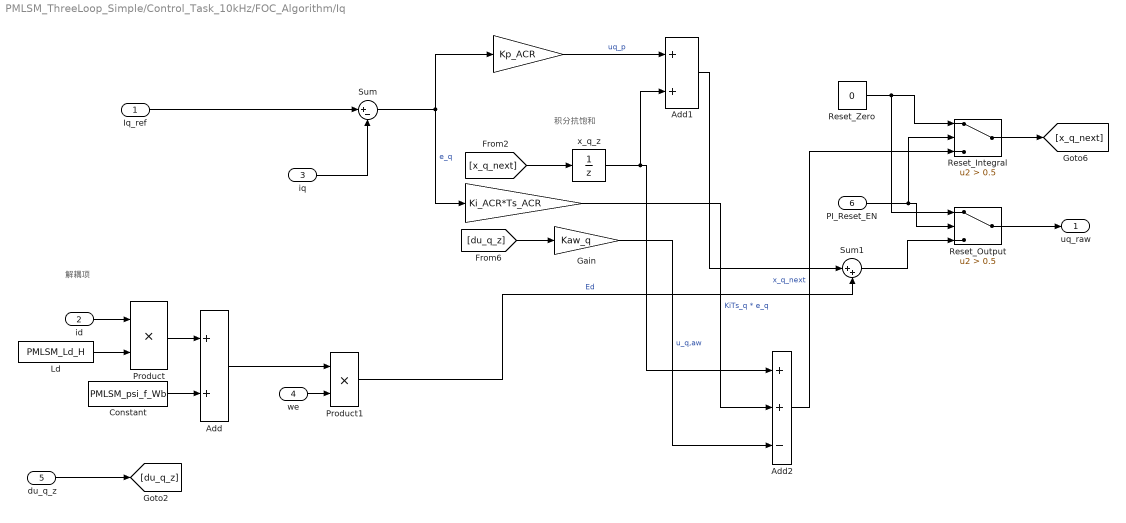
== system PMLSM_ThreeLoop_Simple/Control_Task_10kHz/FOC_Algorithm/Iq ==
  note: 积分抗饱和
  note: 解耦项
  Iq_ref : Inport
  id : Inport  Port=2
  iq : Inport  Port=3
  we : Inport  Port=4
  du_q_z : Inport  Port=5
  PI_Reset_EN : Inport  Port=6
  " " : Gain  Gain=Ki_ACR*Ts_ACR
  "  " : Gain  Gain=Kp_ACR
  Add : Sum
  Add1 : Sum
  Add2 : Sum  Inputs=++-
  Constant : Constant  Value=PMLSM_psi_f_Wb
  Gain : Gain  Gain=Kaw_q
  Ld : Constant  Value=PMLSM_Ld_H
  Product : Product
  Product1 : Product
  Reset_Integral : Switch  Criteria=u2 > Threshold  Threshold=0.5  SaturateOnIntegerOverflow=off  InputSameDT=off
  Reset_Output : Switch  Criteria=u2 > Threshold  Threshold=0.5  SaturateOnIntegerOverflow=off  InputSameDT=off
  Reset_Zero : Constant  Value=0
  Sum : Sum  Inputs=|+-
  Sum1 : Sum  Inputs=|++
  x_q_z : UnitDelay  SampleTime=-1
  uq_raw : Outport
  wires:
  Iq_ref/1 -> Sum/1
  [x_q_next] -> x_q_z/1
  [du_q_z] -> Gain/1
  du_q_z/1 -> [du_q_z]
  "  "/1 -> Add1/1  "uq_p"
  Sum/1 -> " "/1, "  "/1  "e_q"
  Add/1 -> Product1/1
  Constant/1 -> Add/2
  Product/1 -> Add/1
  Ld/1 -> Product/2
  id/1 -> Product/1
  iq/1 -> Sum/2
  we/1 -> Product1/2
  Reset_Output/1 -> uq_raw/1
  Reset_Integral/1 -> [x_q_next]
  PI_Reset_EN/1 -> Reset_Output/2, Reset_Integral/2
  Reset_Zero/1 -> Reset_Output/1, Reset_Integral/1
  Add2/1 -> Reset_Integral/3  "x_q_next"
  Sum1/1 -> Reset_Output/3
  x_q_z/1 -> Add2/1, Add1/2
  " "/1 -> Add2/2  "KiTs_q * e_q"
  Gain/1 -> Add2/3  "u_q,aw"
  Add1/1 -> Sum1/1
  Product1/1 -> Sum1/2  "Ed"

== system PMLSM_ThreeLoop_Simple/Control_Task_10kHz/FOC_Algorithm/SVPWMG ==
  Valpha : Inport
  Vbeta : Inport  Port=2
  Duty Calculate : Subsystem  TreatAsAtomicUnit=on  RTWFcnName=Duty_Caculate_Fun
      settings: RTWFcnNameOpts=User specified
  Sector Caculate : Subsystem  TreatAsAtomicUnit=on  RTWFcnName=Sector_Caculate_Fun
      settings: RTWFcnNameOpts=User specified
  T1T2 Calculate : Subsystem  TreatAsAtomicUnit=on  RTWFcnName=T1T2Caculate_Fun
      settings: RTWFcnNameOpts=User specified
  Udc : Constant  Value=Udc
  XYZ Calculate : Subsystem  TreatAsAtomicUnit=on  RTWFcnName=XYZ_Caculate_Fun
      settings: RTWFcnNameOpts=User specified
  Duty_A : Outport
  Duty_B : Outport  Port=2
  Duty_C : Outport  Port=3
  "N " : Outport  Port=4
  wires:
  Duty Calculate/3(Duty_W) -> Duty_C/1
  Duty Calculate/2(Duty_V) -> Duty_B/1
  Duty Calculate/1(Duty_U) -> Duty_A/1
  XYZ Calculate/3(Z) -> T1T2 Calculate/4(Z)
  XYZ Calculate/2(Y) -> T1T2 Calculate/3(Y)
  XYZ Calculate/1(X) -> T1T2 Calculate/2(X)
  Udc/1 -> XYZ Calculate/3(Udc)
  Sector Caculate/1("N ") -> T1T2 Calculate/1(N), Duty Calculate/1(N), "N "/1
  T1T2 Calculate/2(T2) -> Duty Calculate/3(T2)
  Valpha/1 -> XYZ Calculate/1(Ualpha), Sector Caculate/1(Ualpha)
  T1T2 Calculate/1(T1) -> Duty Calculate/2(T1)
  Vbeta/1 -> XYZ Calculate/2(Ubeta), Sector Caculate/2(Ubeta)

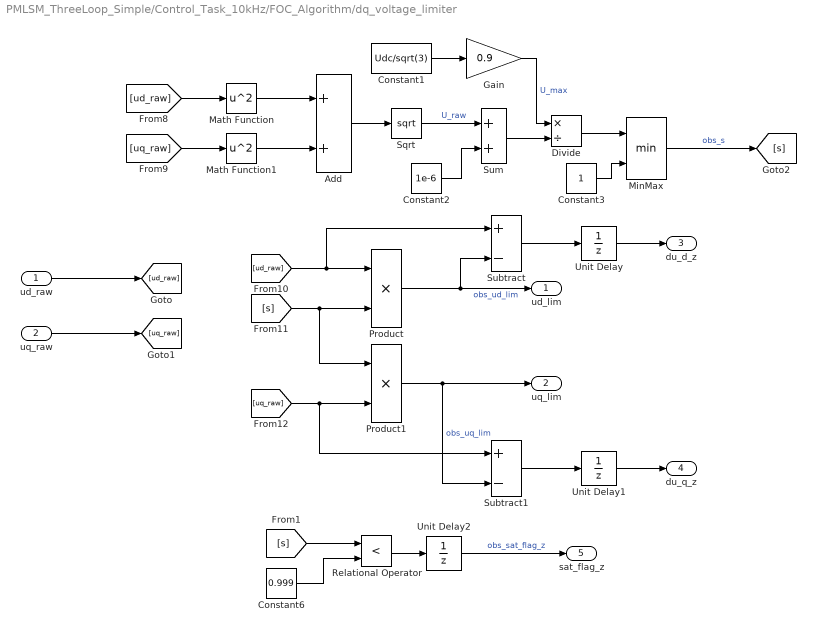
== system PMLSM_ThreeLoop_Simple/Control_Task_10kHz/FOC_Algorithm/dq_voltage_limiter ==
  ud_raw : Inport
  uq_raw : Inport  Port=2
  Add : Sum
  Constant1 : Constant  Value=Udc/sqrt(3)  OutDataTypeStr=double
  Constant2 : Constant  Value=1e-6  OutDataTypeStr=double
  Constant3 : Constant  OutDataTypeStr=double
  Constant6 : Constant  Value=0.999
  Divide : Product  Inputs=*/  OutDataTypeStr=double
  Gain : Gain  Gain=0.9  OutDataTypeStr=double
  Math Function : Math  Operator=square
  Math Function1 : Math  Operator=square
  MinMax : MinMax  Inputs=2
  Product : Product
  Product1 : Product  OutDataTypeStr=double
  Relational Operator : RelationalOperator  Operator=<  OutDataTypeStr=boolean  RndMeth=Simplest  InputSameDT=off
  Sqrt : Sqrt
  Subtract : Sum  Inputs=+-
  Subtract1 : Sum  Inputs=+-
  Sum : Sum
  Unit Delay : UnitDelay  SampleTime=-1
  Unit Delay1 : UnitDelay  SampleTime=-1
  Unit Delay2 : UnitDelay  SampleTime=-1
  ud_lim : Outport
  uq_lim : Outport  Port=2
  du_d_z : Outport  Port=3
  du_q_z : Outport  Port=4
  sat_flag_z : Outport  Port=5
  wires:
  Unit Delay2/1 -> sat_flag_z/1  "obs_sat_flag_z"
  Relational Operator/1 -> Unit Delay2/1
  [s] -> Relational Operator/1
  Constant6/1 -> Relational Operator/2
  Unit Delay1/1 -> du_q_z/1
  Unit Delay/1 -> du_d_z/1
  uq_raw/1 -> [uq_raw]
  ud_raw/1 -> [ud_raw]
  Subtract1/1 -> Unit Delay1/1
  Subtract/1 -> Unit Delay/1
  [uq_raw] -> Product1/2, Subtract1/1
  Product/1 -> ud_lim/1, Subtract/2  "obs_ud_lim"
  [ud_raw] -> Product/1, Subtract/1
  [s] -> Product/2, Product1/1
  Product1/1 -> Subtract1/2, uq_lim/1  "obs_uq_lim"
  MinMax/1 -> [s]  "obs_s"
  [ud_raw] -> Math Function/1
  [uq_raw] -> Math Function1/1
  Math Function/1 -> Add/1
  Math Function1/1 -> Add/2
  Sqrt/1 -> Sum/1  "U_raw"
  Gain/1 -> Divide/1  "U_max"
  Divide/1 -> MinMax/1
  Constant1/1 -> Gain/1
  Add/1 -> Sqrt/1
  Constant3/1 -> MinMax/2
  Constant2/1 -> Sum/2
  Sum/1 -> Divide/2

== system PMLSM_ThreeLoop_Simple/Control_Task_10kHz/Reference_Manager/v_ref_set_slew_limiter ==
  v_ref_set : Inport
  Add : Sum
  Saturation : Saturate  UpperLimit=v_ref_set_step_up  LowerLimit=-v_ref_set_step_dn
  Subtract : Sum  Inputs=+-
  v_ref_set_lim_z : UnitDelay  SampleTime=-1
  v_ref_set_limited : Outport
  wires:
  v_ref_set_lim_z/1 -> Add/2, Subtract/2
  v_ref_set/1 -> Subtract/1
  Saturation/1 -> Add/1
  Subtract/1 -> Saturation/1
  Add/1 -> v_ref_set_limited/1, v_ref_set_lim_z/1

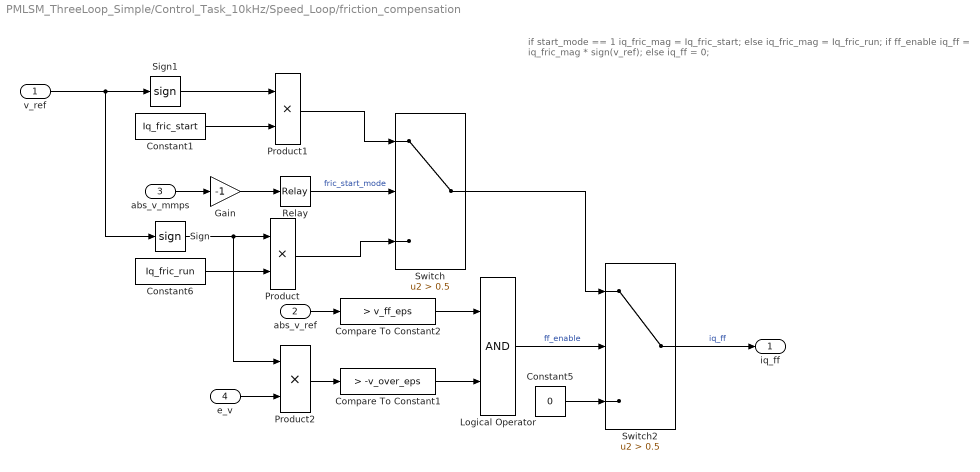
== system PMLSM_ThreeLoop_Simple/Control_Task_10kHz/Speed_Loop/friction_compensation ==
  note: if start_mode == 1
      | 	iq_fric_mag = Iq_fric_start;
      | else
      | 	iq_fric_mag = Iq_fric_run;
      |
      | if ff_enable
      | 	iq_ff = iq_fric_mag * sign(v_ref);
      |  else
      | 	iq_ff = 0;
  v_ref : Inport
  abs_v_ref : Inport  Port=2
  abs_v_mmps : Inport  Port=3
  e_v : Inport  Port=4
  Compare To Constant1 : simulink/Logic and Bit Operations/Compare To Constant  relop=>  const=-v_over_eps  OutDataTypeStr=boolean
  Compare To Constant2 : simulink/Logic and Bit Operations/Compare To Constant  relop=>  const=v_ff_eps  OutDataTypeStr=boolean
  Constant1 : Constant  Value=Iq_fric_start
  Constant5 : Constant  Value=0
  Constant6 : Constant  Value=Iq_fric_run
  Gain : Gain  Gain=-1
  Logical Operator : Logic  AllPortsSameDT=off  OutDataTypeStr=boolean
  Product : Product
  Product1 : Product
  Product2 : Product
  Relay : Relay  OnSwitchValue=-v_stick_on  OffSwitchValue=-v_stick_off
  Sign : Signum
  Sign1 : Signum
  Switch : Switch  Criteria=u2 > Threshold  Threshold=0.5  SaturateOnIntegerOverflow=off  InputSameDT=off
  Switch2 : Switch  Criteria=u2 > Threshold  Threshold=0.5  SaturateOnIntegerOverflow=off  InputSameDT=off
  iq_ff : Outport
  wires:
  v_ref/1 -> Sign/1, Sign1/1
  Sign/1 -> Product2/1, Product/1
  Constant5/1 -> Switch2/3
  Constant6/1 -> Product/2
  abs_v_ref/1 -> Compare To Constant2/1
  Switch2/1 -> iq_ff/1  "iq_ff"
  Switch/1 -> Switch2/1
  Product/1 -> Switch/3
  Sign1/1 -> Product1/1
  Constant1/1 -> Product1/2
  Product1/1 -> Switch/1
  e_v/1 -> Product2/2
  Product2/1 -> Compare To Constant1/1
  Compare To Constant2/1 -> Logical Operator/1
  Compare To Constant1/1 -> Logical Operator/2
  Logical Operator/1 -> Switch2/2  "ff_enable"
  abs_v_mmps/1 -> Gain/1
  Relay/1 -> Switch/2  "fric_start_mode"
  Gain/1 -> Relay/1

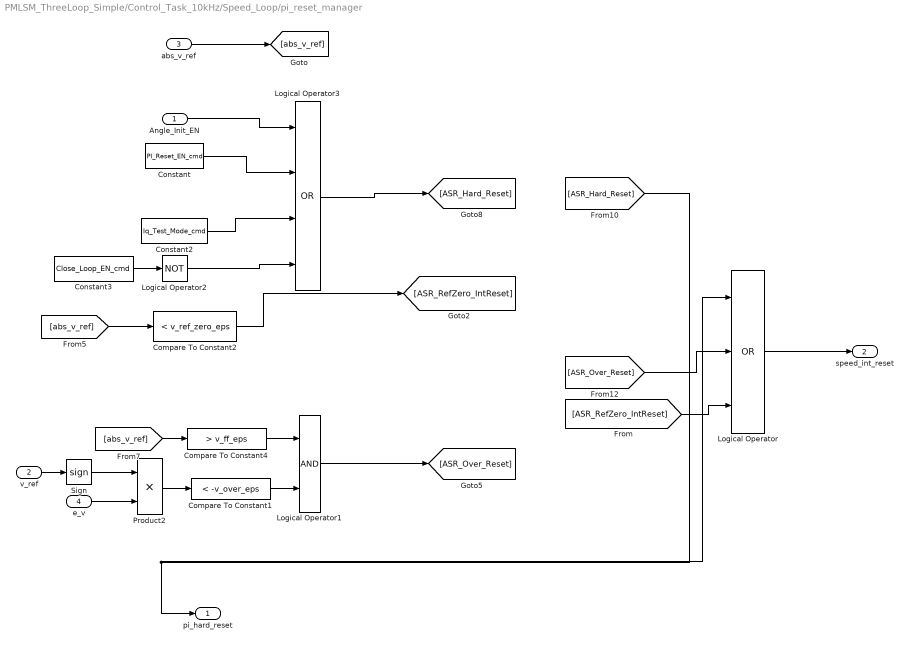
== system PMLSM_ThreeLoop_Simple/Control_Task_10kHz/Speed_Loop/pi_reset_manager ==
  Angle_Init_EN : Inport
  v_ref : Inport  Port=2
  abs_v_ref : Inport  Port=3
  e_v : Inport  Port=4
  Compare To Constant1 : simulink/Logic and Bit Operations/Compare To Constant  relop=<  const=-v_over_eps  OutDataTypeStr=boolean
  Compare To Constant2 : simulink/Logic and Bit Operations/Compare To Constant  relop=<  const=v_ref_zero_eps  OutDataTypeStr=boolean
  Compare To Constant4 : simulink/Logic and Bit Operations/Compare To Constant  relop=>  const=v_ff_eps  OutDataTypeStr=boolean
  Constant : DataStoreRead  DataStoreName=PI_Reset_EN_cmd  IndexOptions=Index vector (dialog)  Indices=1  OutputSizes=1
  Constant2 : DataStoreRead  DataStoreName=Iq_Test_Mode_cmd  IndexOptions=Index vector (dialog)  Indices=1  OutputSizes=1
  Constant3 : DataStoreRead  DataStoreName=Close_Loop_EN_cmd  IndexOptions=Index vector (dialog)  Indices=1  OutputSizes=1
  Logical Operator : Logic  Operator=OR  Inputs=3  AllPortsSameDT=off  OutDataTypeStr=boolean
  Logical Operator1 : Logic  AllPortsSameDT=off  OutDataTypeStr=boolean
  Logical Operator2 : Logic  Operator=NOT  AllPortsSameDT=off  OutDataTypeStr=boolean
  Logical Operator3 : Logic  Operator=OR  Inputs=4  AllPortsSameDT=off  OutDataTypeStr=boolean
  Product2 : Product
  Sign : Signum
  pi_hard_reset : Outport
  speed_int_reset : Outport  Port=2
  wires:
  Compare To Constant2/1 -> [ASR_RefZero_IntReset]
  [abs_v_ref] -> Compare To Constant2/1
  [abs_v_ref] -> Compare To Constant4/1
  e_v/1 -> Product2/2
  Sign/1 -> Product2/1
  Product2/1 -> Compare To Constant1/1
  Compare To Constant1/1 -> Logical Operator1/2
  Compare To Constant4/1 -> Logical Operator1/1
  v_ref/1 -> Sign/1
  abs_v_ref/1 -> [abs_v_ref]
  Logical Operator1/1 -> [ASR_Over_Reset]
  [ASR_RefZero_IntReset] -> Logical Operator/3
  Logical Operator/1 -> speed_int_reset/1
  [ASR_Over_Reset] -> Logical Operator/2
  [ASR_Hard_Reset] -> pi_hard_reset/1, Logical Operator/1
  Logical Operator3/1 -> [ASR_Hard_Reset]
  Angle_Init_EN/1 -> Logical Operator3/1
  Logical Operator2/1 -> Logical Operator3/4
  Constant2/1 -> Logical Operator3/3
  Constant3/1 -> Logical Operator2/1
  Constant/1 -> Logical Operator3/2

== system PMLSM_ThreeLoop_Simple/Inverter_DeadTime/DeadTime_Voltage_Model/Phase_A_DeadTime ==
  duty : Inport
  i_phase : Inport  Port=2
  deadtime_ratio : Inport  Port=3
  vdc : Inport  Port=4
  d_sat : Saturate  UpperLimit=1  LowerLimit=0
  d_sum : Sum  Inputs=+-
  delta_d : Product  Inputs=**
  duty_active_high : Bias  Bias=1  SaturateOnIntegerOverflow=off
  duty_norm : Gain  Gain=-1/PMLSM_pwm_period_counts
  i_deadzone : DeadZone  LowerValue=-PMLSM_deadtime_current_eps_A  UpperValue=PMLSM_deadtime_current_eps_A
  sign_i : Signum
  v0_eff_calc : Product
  v0_eff : Outport
  wires:
  v0_eff_calc/1 -> v0_eff/1  "inv_a_v0_eff"
  vdc/1 -> v0_eff_calc/2
  d_sat/1 -> v0_eff_calc/1  "inv_a_d_eff"
  i_phase/1 -> i_deadzone/1
  duty_norm/1 -> duty_active_high/1
  duty/1 -> duty_norm/1
  duty_active_high/1 -> d_sum/1  "inv_a_d_ideal"
  i_deadzone/1 -> sign_i/1
  sign_i/1 -> delta_d/1  "inv_a_sign_i"
  deadtime_ratio/1 -> delta_d/2
  delta_d/1 -> d_sum/2  "inv_a_delta_d"
  d_sum/1 -> d_sat/1  "inv_a_d_unsat"

== system PMLSM_ThreeLoop_Simple/Inverter_DeadTime/DeadTime_Voltage_Model/Phase_B_DeadTime ==
  duty : Inport
  i_phase : Inport  Port=2
  deadtime_ratio : Inport  Port=3
  vdc : Inport  Port=4
  d_sat : Saturate  UpperLimit=1  LowerLimit=0
  d_sum : Sum  Inputs=+-
  delta_d : Product  Inputs=**
  duty_active_high : Bias  Bias=1  SaturateOnIntegerOverflow=off
  duty_norm : Gain  Gain=-1/PMLSM_pwm_period_counts
  i_deadzone : DeadZone  LowerValue=-PMLSM_deadtime_current_eps_A  UpperValue=PMLSM_deadtime_current_eps_A
  sign_i : Signum
  v0_eff_calc : Product
  v0_eff : Outport
  wires:
  v0_eff_calc/1 -> v0_eff/1  "inv_b_v0_eff"
  vdc/1 -> v0_eff_calc/2
  d_sat/1 -> v0_eff_calc/1  "inv_b_d_eff"
  i_phase/1 -> i_deadzone/1
  duty_norm/1 -> duty_active_high/1
  duty/1 -> duty_norm/1
  duty_active_high/1 -> d_sum/1  "inv_b_d_ideal"
  i_deadzone/1 -> sign_i/1
  sign_i/1 -> delta_d/1  "inv_b_sign_i"
  deadtime_ratio/1 -> delta_d/2
  delta_d/1 -> d_sum/2  "inv_b_delta_d"
  d_sum/1 -> d_sat/1  "inv_b_d_unsat"

== system PMLSM_ThreeLoop_Simple/Inverter_DeadTime/DeadTime_Voltage_Model/Phase_C_DeadTime ==
  duty : Inport
  i_phase : Inport  Port=2
  deadtime_ratio : Inport  Port=3
  vdc : Inport  Port=4
  d_sat : Saturate  UpperLimit=1  LowerLimit=0
  d_sum : Sum  Inputs=+-
  delta_d : Product  Inputs=**
  duty_active_high : Bias  Bias=1  SaturateOnIntegerOverflow=off
  duty_norm : Gain  Gain=-1/PMLSM_pwm_period_counts
  i_deadzone : DeadZone  LowerValue=-PMLSM_deadtime_current_eps_A  UpperValue=PMLSM_deadtime_current_eps_A
  sign_i : Signum
  v0_eff_calc : Product
  v0_eff : Outport
  wires:
  v0_eff_calc/1 -> v0_eff/1  "inv_c_v0_eff"
  vdc/1 -> v0_eff_calc/2
  d_sat/1 -> v0_eff_calc/1  "inv_c_d_eff"
  i_phase/1 -> i_deadzone/1
  duty_norm/1 -> duty_active_high/1
  duty/1 -> duty_norm/1
  duty_active_high/1 -> d_sum/1  "inv_c_d_ideal"
  i_deadzone/1 -> sign_i/1
  sign_i/1 -> delta_d/1  "inv_c_sign_i"
  deadtime_ratio/1 -> delta_d/2
  delta_d/1 -> d_sum/2  "inv_c_delta_d"
  d_sum/1 -> d_sat/1  "inv_c_d_unsat"

== system PMLSM_ThreeLoop_Simple/Control_Task_10kHz/FOC_Algorithm/SVPWMG/Duty Calculate ==
  N : Inport
  T1 : Inport  Port=2
  T2 : Inport  Port=3
  Constant : Constant  Value=Ts
  Fcn : Fcn  Expr=(u[3]-u[1]-u[2])/4
  Fcn1 : Fcn  Expr=(u[3]+u[1]-u[2])/4
  Fcn2 : Fcn  Expr=(u[3]+u[2]+u[1])/4
  Gain : Gain  Gain=CPU_Clock
  Gain1 : Gain  Gain=CPU_Clock
  Gain2 : Gain  Gain=CPU_Clock
  Multiport Switch : MultiPortSwitch  Inputs=6  SaturateOnIntegerOverflow=off  InputSameDT=off
  Multiport Switch1 : MultiPortSwitch  Inputs=6  SaturateOnIntegerOverflow=off  InputSameDT=off
  Multiport Switch2 : MultiPortSwitch  Inputs=6  SaturateOnIntegerOverflow=off  InputSameDT=off
  Mux : Mux  Inputs=3
  Duty_U : Outport
  Duty_V : Outport  Port=2
  Duty_W : Outport  Port=3
  wires:
  Gain2/1 -> Duty_W/1  "DutyW"
  Gain1/1 -> Duty_V/1  "DutyV"
  Gain/1 -> Duty_U/1  "DutyU"
  N/1 -> Multiport Switch/1, Multiport Switch1/1, Multiport Switch2/1
  Fcn2/1 -> Multiport Switch2/4, Multiport Switch2/2, Multiport Switch1/7, Multiport Switch1/3, Multiport Switch/6, Multiport Switch/5
  Fcn1/1 -> Multiport Switch/2, Multiport Switch/7, Multiport Switch1/4, Multiport Switch2/6, Multiport Switch2/3, Multiport Switch1/5
  Fcn/1 -> Multiport Switch1/2, Multiport Switch2/7, Multiport Switch2/5, Multiport Switch1/6, Multiport Switch/4, Multiport Switch/3
  Multiport Switch/1 -> Gain/1
  Multiport Switch1/1 -> Gain1/1
  Multiport Switch2/1 -> Gain2/1
  T1/1 -> Mux/1
  T2/1 -> Mux/2
  Constant/1 -> Mux/3
  Mux/1 -> Fcn1/1, Fcn/1, Fcn2/1

== system PMLSM_ThreeLoop_Simple/Control_Task_10kHz/FOC_Algorithm/SVPWMG/Sector Caculate ==
  Ualpha : Inport
  Ubeta : Inport  Port=2
  B0 : Fcn  Expr=u[2]
  B1 : Fcn  Expr=u[1]*0.866-0.5*u[2]
  B2 : Fcn  Expr=-u[1]*0.866-u[2]*0.5
  Constant : Constant
  Constant1 : Constant  Value=0
  Mux : Mux  Inputs=2
  Mux1 : Mux  Inputs=3
  N : Fcn  Expr=4*u[3]+2*u[2]+u[1]
  Switch : Switch  Criteria=u2 > Threshold  SaturateOnIntegerOverflow=off  InputSameDT=off
  Switch1 : Switch  SaturateOnIntegerOverflow=off  InputSameDT=off
  Switch2 : Switch  Criteria=u2 > Threshold  SaturateOnIntegerOverflow=off  InputSameDT=off
  "N " : Outport  VectorParamsAs1DForOutWhenUnconnected=off
  wires:
  N/1 -> "N "/1  "N"
  Mux1/1 -> N/1
  Switch1/1 -> Mux1/2
  Constant1/1 -> Switch2/3, Switch1/3, Switch/3
  Constant/1 -> Switch1/1, Switch2/1, Switch/1
  B2/1 -> Switch2/2
  B1/1 -> Switch1/2
  B0/1 -> Switch/2
  Mux/1 -> B0/1, B1/1, B2/1
  Ubeta/1 -> Mux/2
  Ualpha/1 -> Mux/1
  Switch/1 -> Mux1/1
  Switch2/1 -> Mux1/3

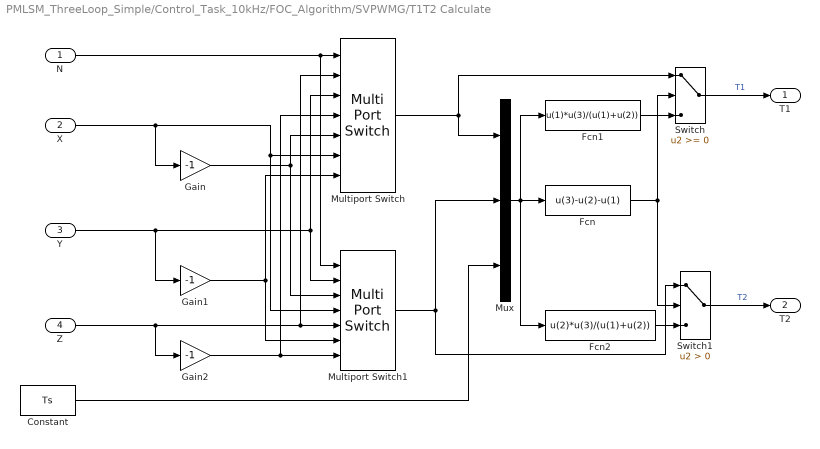
== system PMLSM_ThreeLoop_Simple/Control_Task_10kHz/FOC_Algorithm/SVPWMG/T1T2 Calculate ==
  N : Inport
  X : Inport  Port=2
  Y : Inport  Port=3
  Z : Inport  Port=4
  Constant : Constant  Value=Ts
  Fcn : Fcn  Expr=u(3)-u(2)-u(1)
  Fcn1 : Fcn  Expr=u(1)*u(3)/(u(1)+u(2))
  Fcn2 : Fcn  Expr=u(2)*u(3)/(u(1)+u(2))
  Gain : Gain  Gain=-1
  Gain1 : Gain  Gain=-1
  Gain2 : Gain  Gain=-1
  Multiport Switch : MultiPortSwitch  Inputs=6  SaturateOnIntegerOverflow=off  InputSameDT=off
  Multiport Switch1 : MultiPortSwitch  Inputs=6  SaturateOnIntegerOverflow=off  InputSameDT=off
  Mux : Mux  Inputs=3
  Switch : Switch  SaturateOnIntegerOverflow=off  InputSameDT=off
  Switch1 : Switch  Criteria=u2 > Threshold  SaturateOnIntegerOverflow=off  InputSameDT=off
  T1 : Outport  VectorParamsAs1DForOutWhenUnconnected=off
  T2 : Outport  Port=2  VectorParamsAs1DForOutWhenUnconnected=off
  wires:
  Gain1/1 -> Multiport Switch/7, Multiport Switch1/6
  Gain2/1 -> Multiport Switch1/7, Multiport Switch/4
  Gain/1 -> Multiport Switch/5, Multiport Switch1/3
  X/1 -> Multiport Switch1/4, Multiport Switch/6, Gain/1
  Z/1 -> Gain2/1, Multiport Switch/2, Multiport Switch1/5
  Y/1 -> Gain1/1, Multiport Switch1/2, Multiport Switch/3
  N/1 -> Multiport Switch1/1, Multiport Switch/1
  Multiport Switch1/1 -> Mux/2, Switch1/1
  Multiport Switch/1 -> Mux/1, Switch/1
  Mux/1 -> Fcn2/1, Fcn/1, Fcn1/1
  Fcn/1 -> Switch1/2, Switch/2
  Fcn1/1 -> Switch/3
  Fcn2/1 -> Switch1/3
  Switch/1 -> T1/1  "T1"
  Switch1/1 -> T2/1  "T2"
  Constant/1 -> Mux/3

== system PMLSM_ThreeLoop_Simple/Control_Task_10kHz/FOC_Algorithm/SVPWMG/XYZ Calculate ==
  Ualpha : Inport
  Ubeta : Inport  Port=2
  Udc : Inport  Port=3
  Add : Sum
  Add1 : Sum  Inputs=+-
  Constant1 : Constant  Value=Ts
  Gain : Gain  Gain=3/2
  Gain1 : Gain  Gain=1.7321
  Gain2 : Gain  Gain=0.866
  Math Function : Math  Operator=reciprocal
  Product{,1..3} (4 alike) : Product
  X : Outport
  Y : Outport  Port=2
  Z : Outport  Port=3
  wires:
  Constant1/1 -> Product/1
  Product3/1 -> Y/1  "Y"
  Product2/1 -> Z/1  "Z"
  Add1/1 -> Product2/1
  Add/1 -> Product3/1
  Product1/1 -> X/1  "X"
  Gain/1 -> Add/2, Add1/2
  Gain2/1 -> Add1/1, Add/1
  Product/1 -> Product1/2, Product3/2, Product2/2
  Gain1/1 -> Product1/1
  Ubeta/1 -> Gain1/1, Gain2/1
  Math Function/1 -> Product/2
  Udc/1 -> Math Function/1
  Ualpha/1 -> Gain/1

== matlab function PMLSM_ThreeLoop_Simple/Simple_Host ==
  data: t input; x_ref_mm output; vdc output; load_N output; Close_Loop_EN output; Position_Loop_EN output; PWM_EN output; v_ref_cmd output; id_ref_cmd output; iq_test_mode output; iq_test_ref output; PI_Reset_EN output; Host_Enable_Schedule parameter; Host_Speed_mmps parameter; Host_Id_A parameter; Host_Iq_Test_Mode parameter; Host_Iq_A parameter; Host_PI_Reset_EN parameter; Host_Start_s parameter; Host_Target_mm parameter; Udc parameter; Host_Load_N parameter; Host_Traj_Vmax parameter; Host_Traj_Amax parameter; Host_Traj_Jmax parameter; Host_Speed_Ramp_s parameter
function [x_ref_mm,vdc,load_N,Close_Loop_EN,Position_Loop_EN,PWM_EN,v_ref_cmd,id_ref_cmd,iq_test_mode,iq_test_ref,PI_Reset_EN] = Simple_Host(t, Host_Enable_Schedule, Host_Speed_mmps, Host_Id_A, Host_Iq_Test_Mode, Host_Iq_A, Host_PI_Reset_EN, Host_Start_s, Host_Target_mm, Udc, Host_Load_N, Host_Traj_Vmax, Host_Traj_Amax, Host_Traj_Jmax, Host_Speed_Ramp_s)
% Smooth acceleration - constant speed - smooth deceleration.
x_ref_mm=pmlsm_scurve_profile(t-Host_Start_s,Host_Target_mm,Host_Traj_Vmax,Host_Traj_Amax,Host_Traj_Jmax,Host_Speed_Ramp_s);
r=min(max((t-Host_Start_s)/max(Host_Speed_Ramp_s,1e-6),0),1);
v_ref_cmd=Host_Speed_mmps*(10*r^3-15*r^4+6*r^5);
vdc=Udc; load_N=Host_Load_N;
Close_Loop_EN=0; Position_Loop_EN=0; PWM_EN=0;
for k=1:size(Host_Enable_Schedule,1)
 if t>=Host_Enable_Schedule(k,1)
  Close_Loop_EN=double(Host_Enable_Schedule(k,2)~=0);
  Position_Loop_EN=double(Host_Enable_Schedule(k,3)~=0);
  PWM_EN=double(Host_Enable_Schedule(k,4)~=0);
 end
end
id_ref_cmd=Host_Id_A;
iq_test_mode=Host_Iq_Test_Mode; iq_test_ref=Host_Iq_A;
PI_Reset_EN=Host_PI_Reset_EN;
end
